simulink model "Reaction_Wheels"  (R2021b)
settings: Solver=VariableStepAuto  StartTime=0.0  StopTime=100  RelTol=1e-3
undefined symbols (not defined in the file): A_rw, A_rw_star, omega
libraries: matrix_library x1
settings Model: Creator=jorgemarrero  LastModifiedBy=jorgemarrero

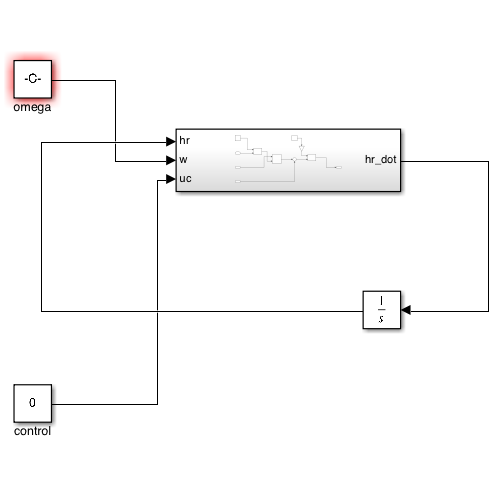
[thumbnail: Simulink's stored preview of the top-level diagram]
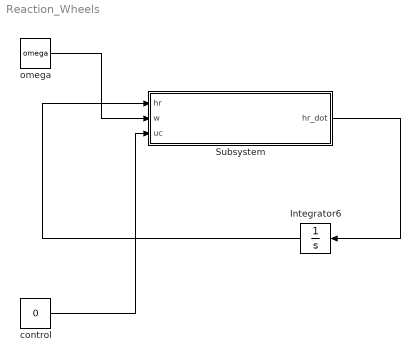
== system Reaction_Wheels ==
  Integrator6 : Integrator  InitialCondition=[0;0;0;0]
  Subsystem : Subsystem
  control : Constant  Value=0
  omega : Constant  Value=omega
  wires:
  Subsystem/1(hr_dot) -> Integrator6/1
  omega/1 -> Subsystem/2(w)
  control/1 -> Subsystem/3(uc)
  Integrator6/1 -> Subsystem/1(hr)

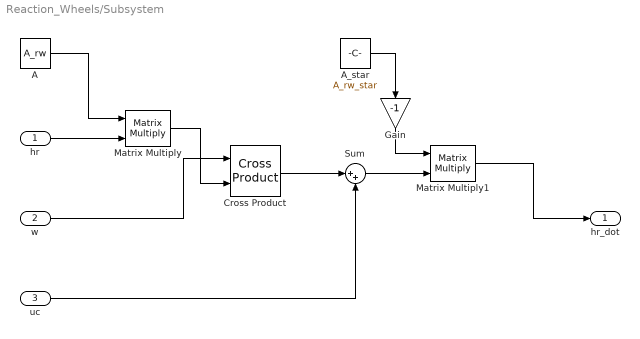
== system Reaction_Wheels/Subsystem ==
  hr : Inport
  w : Inport  Port=2
  uc : Inport  Port=3
  A : Constant  Value=A_rw
  A_star : Constant  Value=A_rw_star
  Cross Product : matrix_library/Cross Product
      settings: SourceProductBaseCode=SL
  Gain : Gain  Gain=-1
  Matrix Multiply : Product  Multiplication=Matrix(*)
  Matrix Multiply1 : Product  Multiplication=Matrix(*)
  Sum : Sum  Inputs=|++
  hr_dot : Outport
  wires:
  hr/1 -> Matrix Multiply/2
  A/1 -> Matrix Multiply/1
  w/1 -> Cross Product/1
  Matrix Multiply/1 -> Cross Product/2
  Cross Product/1 -> Sum/1
  uc/1 -> Sum/2
  Sum/1 -> Matrix Multiply1/2
  A_star/1 -> Gain/1
  Gain/1 -> Matrix Multiply1/1
  Matrix Multiply1/1 -> hr_dot/1
